simulink model "rPIDvsPSO"  (R2014a)
settings: Solver=ode15s  StartTime=0.0  StopTime=1500  MaxStep=1000  RelTol=1e-6
PostLoadFcn:
  | cd(fileparts(which(bdroot)))
undefined symbols (not defined in the file): Kd, Ki, Kp
settings Model: ModifiedByFormat=Mars  ModifiedHistory=Modified by YiXiuKeJi; Taobao is : https://shop197632247.taobao.com  Creator=一休科技  LastModifiedBy=Mars
settings DataIOCC: SignalLoggingSaveFormat=ModelDataLogs  SignalLoggingName=sigsOut
settings OptimizationCC: ExpressionDepthLimit=2147483647  InitFltsAndDblsToZero=on
settings DebuggingCC: SaveWithParameterizedLinksMsg=none  UnderspecifiedInitializationDetection=Classic  SignalResolutionControl=TryResolveAllWithWarning  SolverPrmCheckMsg=none  MultiTaskDSMMsg=warning  MultiTaskCondExecSysMsg=none  FcnCallInpInsideContextMsg=EnableAllAsWarning  FrameProcessingCompatibilityMsg=error  StateNameClashWarn=warning
settings HardwareCC: TargetUnknown=on
settings GRTTargetCC: TargetFcnLib=ansi_tfl_tmw.mat  CombineOutputUpdateFcns=off  GRTInterface=on

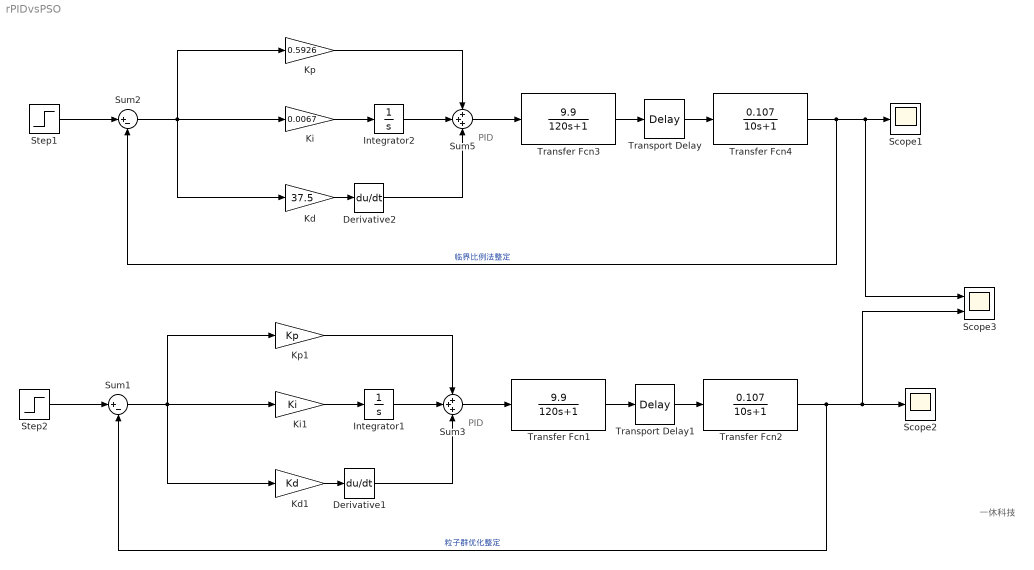
== system rPIDvsPSO ==
  note: PID
  note: PID
  note: 一休科技
  Derivative1 : Derivative
  Derivative2 : Derivative
  Integrator1 : Integrator
  Integrator2 : Integrator
  Kd : Gain  Gain=37.5
  Kd1 : Gain  Gain=Kd
  Ki : Gain  Gain=0.0067
  Ki1 : Gain  Gain=Ki
  Kp : Gain  Gain=0.5926
  Kp1 : Gain  Gain=Kp
  Scope1 : Scope
      settings: TimeRange=auto  MaxDataPoints=5000  SaveToWorkspace=off  YMin=-14.62396  YMax=131.61567  SampleTime=-1
  Scope2 : Scope
      settings: TimeRange=auto  MaxDataPoints=5000  SaveToWorkspace=off  YMin=-12.77653  YMax=114.98877  SampleTime=-1
  Scope3 : Scope  NumInputPorts=2
      settings: TimeRange=auto  ShowLegends=on  MaxDataPoints=5000  SaveToWorkspace=off  SaveName=ScopeData2  YMin=-14.62396~-5  YMax=131.61567~5  SampleTime=-1
  Step1 : Step  Time=0  After=100  SampleTime=0
  Step2 : Step  Time=0  After=100  SampleTime=0
  Sum1 : Sum  Inputs=|+-  SaturateOnIntegerOverflow=on
  Sum2 : Sum  Inputs=|+-  SaturateOnIntegerOverflow=on
  Sum3 : Sum  Inputs=+++
  Sum5 : Sum  Inputs=+++
  Transfer Fcn1 : TransferFcn  Numerator=[9.9 ]  Denominator=[120 1]
  Transfer Fcn2 : TransferFcn  Numerator=[0.107]  Denominator=[10 1]
  Transfer Fcn3 : TransferFcn  Numerator=[9.9 ]  Denominator=[120 1]
  Transfer Fcn4 : TransferFcn  Numerator=[0.107]  Denominator=[10 1]
  Transport Delay : TransportDelay  DelayTime=80
  Transport Delay1 : TransportDelay  DelayTime=80
  wires:
  Derivative2/1 -> Sum5/3
  Integrator2/1 -> Sum5/2
  Sum2/1 -> Kd/1, Kp/1, Ki/1
  Sum5/1 -> Transfer Fcn3/1
  Ki/1 -> Integrator2/1
  Transfer Fcn4/1 -> Scope3/1, Scope1/1, Sum2/2  "临界比例法整定"
  Step1/1 -> Sum2/1
  Transfer Fcn3/1 -> Transport Delay/1
  Transport Delay/1 -> Transfer Fcn4/1
  Kd/1 -> Derivative2/1
  Kp/1 -> Sum5/1
  Transport Delay1/1 -> Transfer Fcn2/1
  Step2/1 -> Sum1/1
  Sum1/1 -> Kd1/1, Kp1/1, Ki1/1
  Ki1/1 -> Integrator1/1
  Transfer Fcn2/1 -> Scope3/2, Scope2/1, Sum1/2  "粒子群优化整定"
  Transfer Fcn1/1 -> Transport Delay1/1
  Sum3/1 -> Transfer Fcn1/1
  Derivative1/1 -> Sum3/3
  Kp1/1 -> Sum3/1
  Integrator1/1 -> Sum3/2
  Kd1/1 -> Derivative1/1
